simulink model "ALU"  (R2018a)
settings: Solver=VariableStepAuto  StartTime=0.0  StopTime=10.0  RelTol=1e-3
settings Model: Creator=midog  LastModifiedBy=midog

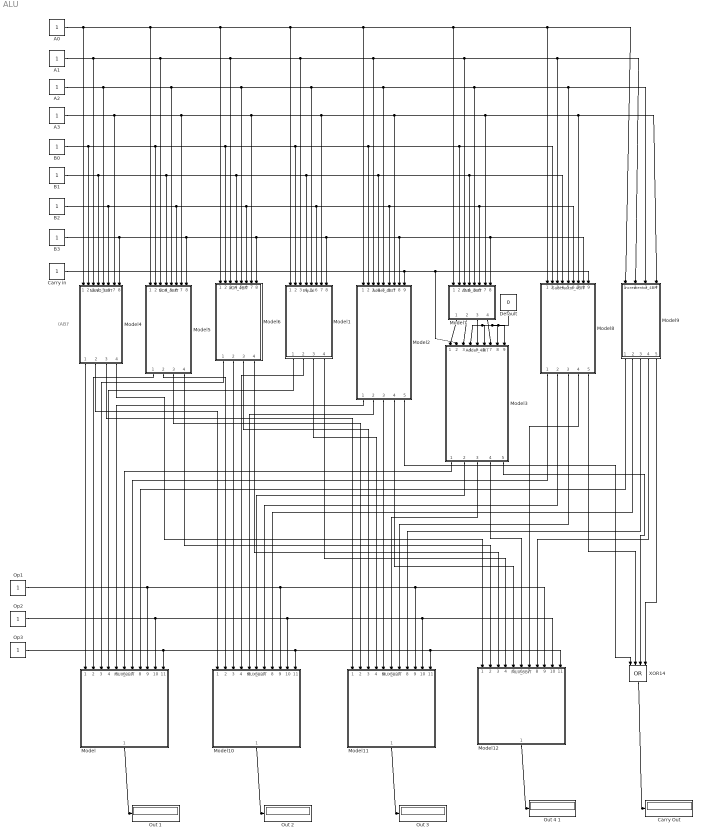
== system ALU ==
  note: (AB)'
  A{0..3} (4 alike) : Constant  OutDataTypeStr=boolean
  B{0..3} (4 alike) : Constant  OutDataTypeStr=boolean
  Carry Out : Display
  Carry in : Constant  OutDataTypeStr=boolean
  Default : Constant  Value=0  OutDataTypeStr=boolean
  Model{,10..12} (4 alike) : ModelReference  ModelNameDialog=MUX_8BIT.slx  SimulationMode=Normal  ModelReferenceVersion=1.1
  Model1 : ModelReference  ModelNameDialog=Equal.slx  SimulationMode=Normal  ModelReferenceVersion=1.2
  Model2 : ModelReference  ModelNameDialog=Adder_4BIT.slx  SimulationMode=Normal  ModelReferenceVersion=1.4
  Model3 : ModelReference  ModelNameDialog=Adder_4BIT.slx  SimulationMode=Normal  ModelReferenceVersion=1.4
  Model4 : ModelReference  ModelNameDialog=NAND_4BIT.slx  SimulationMode=Normal  ModelReferenceVersion=1.1
  Model5 : ModelReference  ModelNameDialog=NOR_4BIT.slx  SimulationMode=Normal  ModelReferenceVersion=1.1
  Model6 : ModelReference  ModelNameDialog=XOR_4BIT.slx  SimulationMode=Normal  ModelReferenceVersion=1.1
  Model7 : ModelReference  ModelNameDialog=AND_4BIT.slx  SimulationMode=Normal  ModelReferenceVersion=1.1
  Model8 : ModelReference  ModelNameDialog=Subtractor_4BIT.slx  SimulationMode=Normal  ModelReferenceVersion=1.2
  Model9 : ModelReference  ModelNameDialog=Incrementor_4BIT.slx  SimulationMode=Normal  ModelReferenceVersion=1.1
  "Op1 " : Constant  OutDataTypeStr=boolean
  Op2 : Constant  OutDataTypeStr=boolean
  Op3 : Constant  OutDataTypeStr=boolean
  "Out 1 " : Display
  Out 2 : Display
  Out 3 : Display
  Out 4 1 : Display
  XOR14 : Logic  Operator=OR  Inputs=4  IconShape=distinctive  AllPortsSameDT=off  OutDataTypeStr=boolean
  wires:
  A0/1 -> Model4/1, Model6/1, Model1/1, Model2/1, Model9/1, Model8/1, Model7/1, Model5/1
  A1/1 -> Model4/3, Model6/3, Model1/3, Model2/3, Model9/2, Model8/3, Model7/3, Model5/3
  A2/1 -> Model4/5, Model6/5, Model1/5, Model2/5, Model9/3, Model8/5, Model7/5, Model5/5
  A3/1 -> Model4/7, Model6/7, Model1/7, Model2/7, Model7/7, Model9/4, Model8/7, Model5/7
  B0/1 -> Model4/2, Model6/2, Model1/2, Model2/2, Model7/2, Model8/2, Model5/2
  B1/1 -> Model4/4, Model6/4, Model1/4, Model2/4, Model8/4, Model7/4, Model5/4
  B2/1 -> Model4/6, Model6/6, Model1/6, Model2/6, Model8/6, Model7/6, Model5/6
  Carry in/1 -> Model8/9, Model3/2, Model2/9
  Model7/1 -> Model3/1
  Model7/2 -> Model3/3
  Model7/3 -> Model3/5
  Model7/4 -> Model3/7
  Default/1 -> Model3/8, Model3/6, Model3/4, Model3/9
  B3/1 -> Model4/8, Model6/8, Model1/8, Model2/8, Model8/8, Model7/8, Model5/8
  Model4/1 -> Model/1
  Model5/1 -> Model/2
  Model6/1 -> Model/3
  Model1/1 -> Model/4
  Model2/1 -> Model/5
  Model3/1 -> Model/6
  Model8/1 -> Model/7
  Model9/1 -> Model/8
  Model4/2 -> Model10/1
  Model5/2 -> Model10/2
  Model6/2 -> Model10/3
  Model1/2 -> Model10/4
  Model2/2 -> Model10/5
  Model3/2 -> Model10/6
  Model8/2 -> Model10/7
  Model9/2 -> Model10/8
  Model4/3 -> Model11/1
  Model5/3 -> Model11/2
  Model6/3 -> Model11/3
  Model1/3 -> Model11/4
  Model2/3 -> Model11/5
  Model3/3 -> Model11/6
  Model8/3 -> Model11/7
  Model9/3 -> Model11/8
  Model4/4 -> Model12/1
  Model5/4 -> Model12/2
  Model6/4 -> Model12/3
  Model1/4 -> Model12/4
  Model2/4 -> Model12/5
  Model3/4 -> Model12/6
  Model8/4 -> Model12/7
  Model9/4 -> Model12/8
  Op2/1 -> Model12/10, Model11/10, Model10/10, Model/10
  Op3/1 -> Model/11, Model11/11, Model12/11, Model10/11
  "Op1 "/1 -> Model/9, Model12/9, Model11/9, Model10/9
  Model/1 -> "Out 1 "/1
  Model10/1 -> Out 2/1
  Model11/1 -> Out 3/1
  Model12/1 -> Out 4 1/1
  Model2/5 -> XOR14/1
  Model8/5 -> XOR14/2
  Model3/5 -> XOR14/3
  Model9/5 -> XOR14/4
  XOR14/1 -> Carry Out/1
